simulink model "Junctions6_tmp"  (Simulink 8.3)
settings: Solver=ode45  StartTime=0.0  StopTime=10.0  RelTol=1e-3
settings Model: Creator=scaife  LastModifiedBy=bourbouh  CovSFcnEnable=on  ExtModeAutoUpdateStatusClock=off
settings DataIOCC: SignalLoggingName=sigsOut
settings DebuggingCC: SaveWithParameterizedLinksMsg=none  SignalResolutionControl=TryResolveAllWithWarning  SolverPrmCheckMsg=none  MultiTaskDSMMsg=warning  MultiTaskCondExecSysMsg=none  FrameProcessingCompatibilityMsg=error  StateNameClashWarn=none  StrictBusMsg=None
settings HardwareCC: TargetUnknown=on
settings SFSimCC: SimParseCustomCode=off
settings GRTTargetCC: GeneratePreprocessorConditionals=Use local settings

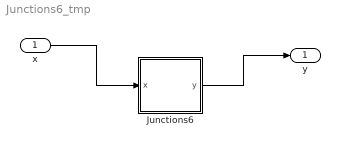
== system Junctions6_tmp ==
  x : Inport
  Junctions6 : Stateflow chart  TreatAsAtomicUnit=on
      settings: PermitHierarchicalResolution=ParametersOnly
  y : Outport
  wires:
  x/1 -> Junctions6/1(x)
  Junctions6/1(y) -> y/1

== stateflow chart Junctions6 ==
  state TOP
    state A
    state B
    state C
    state D
    (default) -> A [order 1] : [x<4]{y+=1}
    (default) -> B [order 2] : [x>=4]{y+=10}
    A -> (junction 8) : [x<=2]{y+=100}
    B -> (junction 8) : [x>=6]{y+=1000}
    (junction 8) -> D [order 1] : [x %% 3 == 0]{y+=100000}
    (junction 8) -> C [order 2] : [x %% 3 == 1]{y+=10000}
    D -> C
    C -> TOP
  (default) -> TOP
  data: x input int32; y output int32 =111111
